simulink model "DCMotor"  (R2017a)
settings: Solver=VariableStepAuto  StartTime=0.0  StopTime=1  RelTol=1e-3
values from neighbouring files (symbols this model uses):
  b = 0.1    [DCMotVal.mat]
  J = 0.01    [DCMotVal.mat]
  K = 0.01    [DCMotVal.mat]
  L = 0.5    [DCMotVal.mat]
  R = 1    [DCMotVal.mat]
settings Model: Creator=Igor Khimchenko  LastModifiedBy=Igor Khimchenko

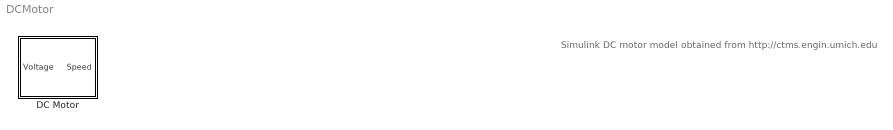
== system DCMotor ==
  note: Simulink DC motor model obtained from http://ctms.engin.umich.edu
  DC Motor : Subsystem

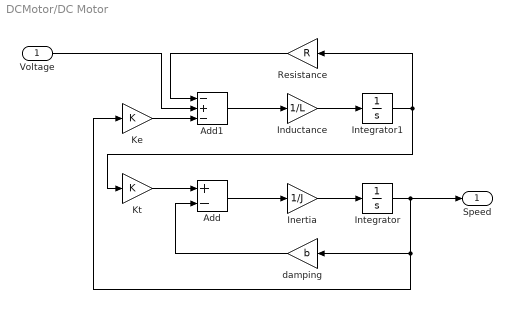
== system DCMotor/DC Motor ==
  Voltage : Inport
  Add : Sum  Inputs=+-
  Add1 : Sum  Inputs=-+-
  Inductance : Gain  Gain=1/L
  Inertia : Gain  Gain=1/J
  Integrator : Integrator
  Integrator1 : Integrator
  Ke : Gain  Gain=K
  Kt : Gain  Gain=K
  Resistance : Gain  Gain=R
  damping : Gain  Gain=b
  Speed : Outport
  wires:
  Resistance/1 -> Add1/1
  Inductance/1 -> Integrator1/1
  Kt/1 -> Add/1
  Ke/1 -> Add1/3
  Inertia/1 -> Integrator/1
  Add1/1 -> Inductance/1
  Integrator/1 -> Ke/1, damping/1, Speed/1
  damping/1 -> Add/2
  Voltage/1 -> Add1/2
  Integrator1/1 -> Resistance/1, Kt/1
  Add/1 -> Inertia/1
